simulink model "third_task"  (R2023a)
settings: Solver=VariableStepAuto  StartTime=0.0  StopTime=100  RelTol=1e-3
undefined symbols (not defined in the file): axang2rotm, j, K, k_phi, k_w, m, n, nd, q0, vs_des
settings Model: Creator=Nabil Samaan  LastModifiedBy=dvogureckiy99
settings DebuggingCC: UnconnectedInputMsg=warning  UnconnectedOutputMsg=warning  UnconnectedLineMsg=warning
settings ModelReferenceCC: EnableRefExpFcnMdlSchedulingChecks=on
settings RTWCC: DLArmComputeVersion=19.05

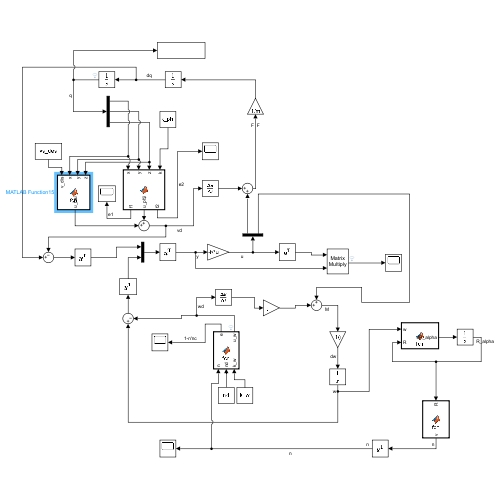
[thumbnail: Simulink's stored preview of the top-level diagram]
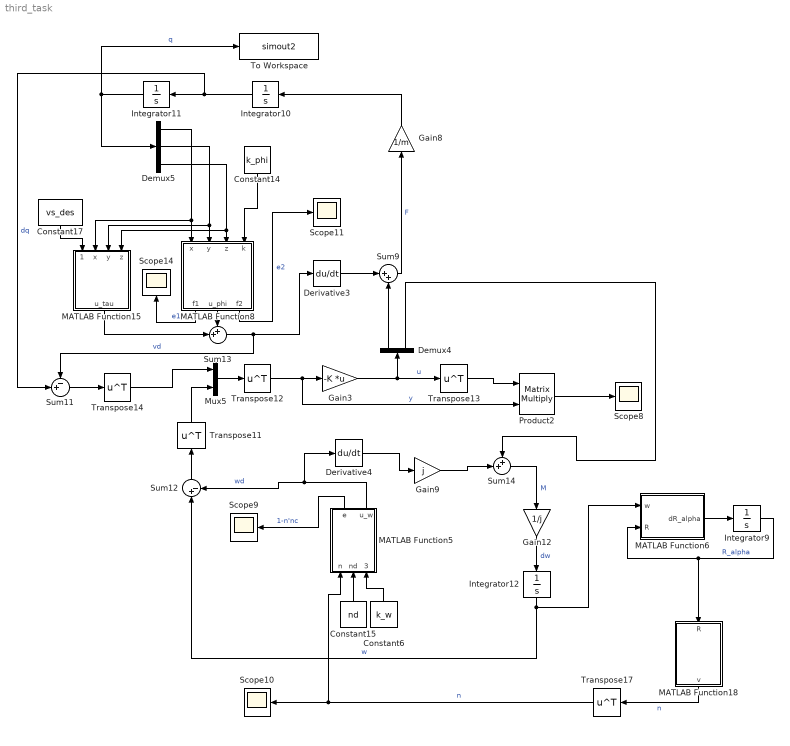
== system third_task ==
  Constant14 : Constant  Value=k_phi
  Constant15 : Constant  Value=nd
  Constant17 : Constant  Value=vs_des
  Constant6 : Constant  Value=k_w
  Demux4 : Demux  Outputs=2
  Demux5 : Demux  Outputs=3
  Derivative3 : Derivative  CoefficientInTFapproximation=10
  Derivative4 : Derivative
  Gain12 : Gain  Gain=1/j
  Gain3 : Gain  Gain=-K  Multiplication=Matrix(K*u)
  Gain8 : Gain  Gain=1/m
  Gain9 : Gain  Gain=j
  Integrator10 : Integrator  InitialCondition=[0;0;0]
  Integrator11 : Integrator  InitialCondition=q0
  Integrator12 : Integrator  InitialCondition=[0;0;0]
  Integrator9 : Integrator  InitialCondition=axang2rotm([n' / norm(n) , norm(n)])
  MATLAB Function15 : MATLAB Function  TreatAsAtomicUnit=on
  MATLAB Function18 : MATLAB Function  TreatAsAtomicUnit=on
  MATLAB Function5 : MATLAB Function  TreatAsAtomicUnit=on
  MATLAB Function6 : MATLAB Function  TreatAsAtomicUnit=on
  MATLAB Function8 : MATLAB Function  TreatAsAtomicUnit=on
  Mux5 : Mux  Inputs=2
  Product2 : Product  Multiplication=Matrix(*)
  Scope{8..11,14} (5 alike) : Scope
  Sum11 : Sum  Inputs=-+|
  Sum12 : Sum  Inputs=|+-
  Sum13 : Sum  Inputs=++|
  Sum14 : Sum  Inputs=++|
  Sum9 : Sum  Inputs=|++
  To Workspace : ToWorkspace  VariableName=simout2  SaveFormat=Timeseries  SampleTime=-1
  Transpose{11..14,17} (5 alike) : Math  Operator=transpose
  wires:
  MATLAB Function6/1(dR_alpha) -> Integrator9/1
  Constant17/1 -> MATLAB Function15/1(vs_des)
  Sum13/1 -> Sum11/1, Derivative3/1  "vd"
  Integrator11/1 -> Demux5/1, To Workspace/1  "q"
  Constant15/1 -> MATLAB Function5/2(nd)
  Demux5/2 -> MATLAB Function15/3(y), MATLAB Function8/2(y)
  Demux5/3 -> MATLAB Function15/4(z), MATLAB Function8/3(z)
  MATLAB Function5/2(u_w) -> Derivative4/1, Sum12/2  "wd"
  Gain12/1 -> Integrator12/1  "dw"
  Sum14/1 -> Gain12/1  "M"
  Mux5/1 -> Transpose12/1
  Constant14/1 -> MATLAB Function8/4(k)
  Transpose13/1 -> Product2/1
  Derivative3/1 -> Sum9/1
  Demux5/1 -> MATLAB Function15/2(x), MATLAB Function8/1(x)
  Sum9/1 -> Gain8/1  "F"
  Product2/1 -> Scope8/1
  MATLAB Function5/1(e) -> Scope9/1  "1-n'nc"
  Gain9/1 -> Sum14/2
  Integrator12/1 -> MATLAB Function6/1(w), Sum12/1  "w"
  MATLAB Function8/2(u_phi) -> Sum13/1
  Integrator10/1 -> Sum11/2, Integrator11/1  "dq"
  Constant6/1 -> MATLAB Function5/3(k_w)
  MATLAB Function15/1(u_tau) -> Sum13/2
  Transpose11/1 -> Mux5/2
  Sum12/1 -> Transpose11/1
  Transpose12/1 -> Product2/2, Gain3/1  "y"
  Sum11/1 -> Transpose14/1
  Transpose14/1 -> Mux5/1
  Gain3/1 -> Transpose13/1, Demux4/1  "u"
  Derivative4/1 -> Gain9/1
  Integrator9/1 -> MATLAB Function18/1(R), MATLAB Function6/2(R)  "R_alpha"
  Transpose17/1 -> Scope10/1, MATLAB Function5/1(n)  "n"
  MATLAB Function8/3(f2) -> Scope11/1  "e2"
  MATLAB Function8/1(f1) -> Scope14/1  "e1"
  Demux4/2 -> Sum14/1
  MATLAB Function18/1(v) -> Transpose17/1  "n"
  Demux4/1 -> Sum9/2
  Gain8/1 -> Integrator10/1

== matlab function third_task/MATLAB Function6 ==
  data: w input; dR_alpha output; R input
function dR_alpha= fcn(w,R)


s=[0 w(3) -w(2);-w(3) 0 w(1);w(2) -w(1) 0];

dR_alpha=s*R;

== matlab function third_task/MATLAB Function15 ==
  data: vs_des input; x input; u_tau output; y input; z input
function u_tau= fcn(vs_des,x,y,z)

gf1=[0.28*x;0.96*y;0];
gf2=[0;0.66*y;1];
c=cross(gf1,gf2);
j1=c/norm(c);
j2=gf1/norm(gf1);
j3=gf2/norm(gf2);

J=[j1';j2';j3'];
j_inv=J^(-1);

u_tau=j_inv*[vs_des;0;0];

== matlab function third_task/MATLAB Function5 ==
  data: e output; n input; u_w output; nd input; k_w input
function [e,u_w]= fcn(n,nd,k_w)

s=[0 nd(3) -nd(2);-nd(3) 0 nd(1);nd(2) -nd(1) 0];
e=1-((n')*nd);

u_w=-s*n*k_w*e;

== matlab function third_task/MATLAB Function8 ==
  data: f1 output; u_phi output; f2 output; x input; y input; z input; k input
function[f1,u_phi,f2]= fcn(x,y,z,k)

f1= 0.14*x^2 +0.48*y^2 -225;

gf1=[0.28*x;0.96*y;0];


f2=z+0.33*y^2 -3;

gf2=[0;0.66*y;1];

u_phi=-k*(f1*gf1+f2*gf2);

== matlab function third_task/MATLAB Function18 ==
  data: v output; R input
function v= fcn(R)

p = rotm2axang(R);
v = p(1:3)*p(4);
